simulink library "libAeroLookUpTables"  (R2020b)
settings: Solver=VariableStepAuto  StartTime=0.0  StopTime=10.0  RelTol=1e-3
undefined symbols (not defined in the file): data, table
settings Model: Creator=caatay  LastModifiedBy=caatay

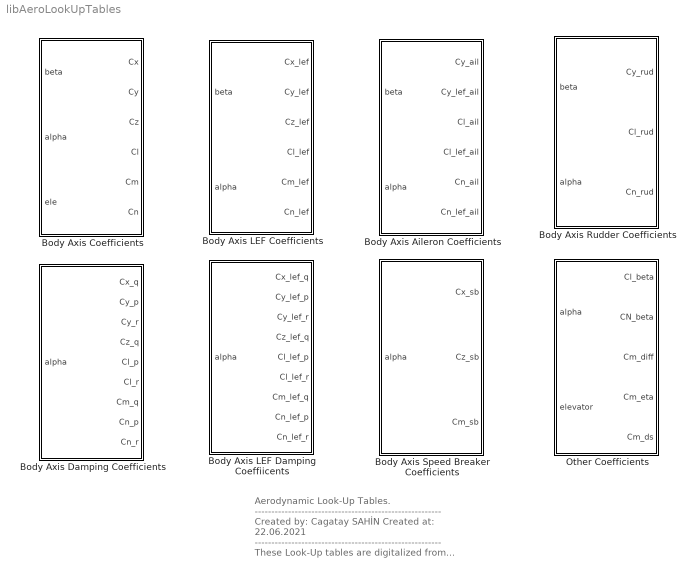
== system libAeroLookUpTables ==
  note: Aerodynamic Look-Up Tables.
      | --------------------------------------------------------
      | Created by: Cagatay SAHİN
      | Created at: 22.06.2021
      | --------------------------------------------------------
      | These Look-Up tables are digitalized from
      | Nguyen's NASA works.
      | The reference article can be found in
      | "references folder".
      | --------------------------------------------------------
      | for question:
      | cagataysahin44@gmail.com
  Body Axis Aileron Coefficients : Subsystem  mask(Aerodynamic Model - Look-Up Tables - Body Axis Aileron Aerodynamic Data){data=data}
      mask prompts: data "Aerodynamic Look-Up Table Data"
      mask help: 2-D Body axis aerodynamic look-up tables, effect on aileron deflection, to obtain that aerodynamic coefficients with using linear interpolation methods.
      mask Help:
      | This block calculates body axis aileron aerodynamic coefficient with using interpolation method.
      | According to reference, all look-up tables are 2-dimension.
      | -------------------------------------------------------------------------------------------------------------------------------------------------
      | Inputs of this block set are;
      | 	alpha = Angle of attack value that comes from equation of motion or frame transformation. [deg]
      | 	beta = Sideslip angle value that comes from equation of motion or frame transformation. [deg]
      | Output of this block set is;
      | 	C_{i_{ail}} = Body axis coefficients for instance Cx_rud, Cy_rud Cz_rud... .
      | -------------------------------------------------------------------------------------------------------------------------------------------------
      | Look-up tables are obtained from Nguyen's work. Reference can be found in "literature" subfolder.
      | For question: "cagataysahin44@gmail.com"
      mask Display:
      | port_label('input',1,'\beta','texmode','on');
      | port_label('input',2,'\alpha','texmode','on');
      | 
      | port_label('output',1,'C_{y_{ail}}','texmode','on');
      | port_label('output',2,'C_{y_{lef_{ail}}}','texmode','on');
      | port_label('output',3,'C_{l_{ail}}','texmode','on');
      | port_label('output',4,'C_{l_{lef_{ail}}}','texmode','on');
      | port_label('output',5,'C_{n_{ail}}','texmode','on');
      | port_label('output',6,'C_{n_{lef_{ail}}}','texmode','on');
  Body Axis Coefficients : Subsystem  mask(Aerodynamic Model - Look-Up Tables - Body Axis Aerodynamic Data){data=data}
      mask prompts: data "Aerodynamic Look-up Table Data"
      mask help: 3-D body axis aerodynamic look-up tables to obtain body axis aerodynamic coefficients with using interpolation method.
      mask Help:
      | This block calculates body axis aerodynamic coefficient with using interpolation method.
      | According to reference, all look-up tables are 3-dimension except "CY".
      | -------------------------------------------------------------------------------------------------------------------------------------------------
      | Inputs of this block set are;
      | 	alpha = Angle of attack value that comes from equation of motion or frame transformation. [deg]
      | 	beta = Sideslip angle value that comes from equation of motion or frame transformation. [deg]
      | 	elevator = Actuated elevator deflection value that comes from actuator. [deg]
      | Output of this block set is;
      | 	C_{i} = Body axis coefficients for instance Cx, Cy, Cz ... .
      | -------------------------------------------------------------------------------------------------------------------------------------------------
      | Look-up tables are obtained from Nguyen's work. Reference can be found in "literature" subfolder.
      | For question: "cagataysahin44@gmail.com"
      mask Display:
      | port_label('input',1,'\beta','texmode','on');
      | port_label('input',2,'\alpha','texmode','on');
      | port_label('input',3,'\delta_{el}','texmode','on');
      | 
      | port_label('output',1,'C_{x}','texmode','on');
      | port_label('output',2,'C_{y}','texmode','on');
      | port_label('output',3,'C_{z}','texmode','on');
      | port_label('output',4,'C_{l}','texmode','on');
      | port_label('output',5,'C_{m}','texmode','on');
      | port_label('output',6,'C_{n}','texmode','on');
  Body Axis Damping Coefficients : Subsystem  mask(Aerodynamic Model - Look-Up Tables - Body Axis Damping Aerodynamic Data){data=data}
      mask prompts: data "Aerodynamic Look-Up Table Data"
      mask help: 1-D Body axis damping aerodynamic look-up tables to obtain body axis damping aerodynamic coefficients with using interpolation method.
      mask Help:
      | This block calculates body axis aerodynamic coefficient with using interpolation method.
      | According to reference, all look-up tables are 1-dimension
      | -------------------------------------------------------------------------------------------------------------------------------------------------
      | Inputs of this block set are;
      | 	alpha = Angle of attack value that comes from equation of motion or frame transformation. [deg]
      | Output of this block set is;
      | 	C_{i_{j}} = Body axis damping coefficients for instance Cx_q, Cy_p, Cz_q ... .
      | -------------------------------------------------------------------------------------------------------------------------------------------------
      | Look-up tables are obtained from Nguyen's work. Reference can be found in "literature" subfolder.
      | For question: "cagataysahin44@gmail.com"
      mask Display:
      | port_label('input',1,'\alpha','texmode','on');
      | 
      | 
      | port_label('output',1,'C_{x_{q}}','texmode','on');
      | port_label('output',2,'C_{y_{p}}','texmode','on');
      | port_label('output',3,'C_{y_{r}}','texmode','on');
      | port_label('output',4,'C_{z_{q}}','texmode','on');
      | port_label('output',5,'C_{l_{p}}','texmode','on');
      | port_label('output',6,'C_{l_{r}}','texmode','on');
      | port_label('output',7,'C_{m_{q}}','texmode','on');
      | port_label('output',8,'C_{n_{p}}','texmode','on');
      | port_label('output',9,'C_{n_{r}}','texmode','on');
  Body Axis LEF Damping Coeffiicents : Subsystem  mask(Aerodynamic Model - Look-Up Tables - Body Axis LEF Damping Aerodynamic Data){data=data}
      mask prompts: data "Aerodynamic Look-Up Table Data"
      mask help: 1-D Body axis damping aerodynamic look-up tables, effect on leading edge flap deflections, to obtain that aerodynamic coefficient with using interpolation method.
      mask Help:
      | This block calculates body axis LEF aerodynamic coefficient with using interpolation method.
      | According to reference, all look-up tables are 1-dimension
      | -------------------------------------------------------------------------------------------------------------------------------------------------
      | Inputs of this block set are;
      | 	alpha = Angle of attack value that comes from equation of motion or frame transformation. [deg]
      | Output of this block set is;
      | 	C_{i_lef_{j}} = Body axis damping coefficients for instance Cx_lef_q, Cy_lef_p, Cz_lef_q ... .
      | -------------------------------------------------------------------------------------------------------------------------------------------------
      | Look-up tables are obtained from Nguyen's work. Reference can be found in "literature" subfolder.
      | For question: "cagataysahin44@gmail.com"
      mask Display:
      | port_label('input',1,'\alpha','texmode','on');
      | 
      | 
      | port_label('output',1,'C_{x_{lef}_{q}}','texmode','on');
      | port_label('output',2,'C_{y_{lef}_{p}}','texmode','on');
      | port_label('output',3,'C_{y_{lef}_{r}}','texmode','on');
      | port_label('output',4,'C_{z_{lef}_{q}}','texmode','on');
      | port_label('output',5,'C_{l_{lef}_{p}}','texmode','on');
      | port_label('output',6,'C_{l_{lef}_{r}}','texmode','on');
      | port_label('output',7,'C_{m_{lef}_{q}}','texmode','on');
      | port_label('output',8,'C_{n_{lef}_{p}}','texmode','on');
      | port_label('output',9,'C_{n_{lef}_{r}}','texmode','on');
  Body Axis LEF Coefficients : Subsystem  mask(Aerodynamic Model - Look-Up Tables - Body Axis Leading Edge Flap Aerodynamic Data){data=data}
      mask prompts: data "Aerodynamic Look-up Table Data"
      mask help: 2-D body axis aerodynamic look-up tables, effect on leading edge flap deflection, to obtain that aerodynamic coefficients with using linear interpolation methods.
      mask Help:
      | This block calculates body axis LEF aerodynamic coefficient with using interpolation method.
      | According to reference, all look-up tables are 2-dimension.
      | -------------------------------------------------------------------------------------------------------------------------------------------------
      | Inputs of this block set are;
      | 	alpha = Angle of attack value that comes from equation of motion or frame transformation. [deg]
      | 	beta = Sideslip angle value that comes from equation of motion or frame transformation. [deg]
      | Output of this block set is;
      | 	C_{i_{lef}} = Body axis coefficients for instance Cx_lef, Cy_lef, Cz_lef ... .
      | -------------------------------------------------------------------------------------------------------------------------------------------------
      | Look-up tables are obtained from Nguyen's work. Reference can be found in "literature" subfolder.
      | For question: "cagataysahin44@gmail.com"
      mask Display:
      | port_label('input',1,'\beta','texmode','on');
      | port_label('input',2,'\alpha','texmode','on');
      | 
      | port_label('output',1,'C_{x_{lef}}','texmode','on');
      | port_label('output',2,'C_{y_{lef}}','texmode','on');
      | port_label('output',3,'C_{z_{lef}}','texmode','on');
      | port_label('output',4,'C_{l_{lef}}','texmode','on');
      | port_label('output',5,'C_{m_{lef}}','texmode','on');
      | port_label('output',6,'C_{n_{lef}}','texmode','on');
  Body Axis Rudder Coefficients : Subsystem  mask(Aerodynamic Model - Look-Up Tables - Body Axis Rudder Aerodynamic Data){data=data}
      mask prompts: data "Aerodynamic Look-up Table Data"
      mask help: 2-D Body axi aerodynamic look-up tables, effect on rudder deflection, to obtain that aerodynamic coefficients with using linear interpolation methods.
      mask Help:
      | This block calculates body axis rudder aerodynamic coefficient with using interpolation method.
      | According to reference, all look-up tables are 2-dimension.
      | -------------------------------------------------------------------------------------------------------------------------------------------------
      | Inputs of this block set are;
      | 	alpha = Angle of attack value that comes from equation of motion or frame transformation. [deg]
      | 	beta = Sideslip angle value that comes from equation of motion or frame transformation. [deg]
      | Output of this block set is;
      | 	C_{i_{rud}} = Body axis coefficients for instance Cx_rud, Cy_rud Cz_rud... .
      | -------------------------------------------------------------------------------------------------------------------------------------------------
      | Look-up tables are obtained from Nguyen's work. Reference can be found in "literature" subfolder.
      | For question: "cagataysahin44@gmail.com"
      mask Display:
      | port_label('input',1,'\beta','texmode','on');
      | port_label('input',2,'\alpha','texmode','on');
      | 
      | port_label('output',1,'C_{y_{rud}}','texmode','on');
      | port_label('output',2,'C_{l_{rud}}','texmode','on');
      | port_label('output',3,'C_{n_{rud}}','texmode','on');
  Body Axis Speed Breaker Coefficients : Subsystem  mask(Aerodynamic Model - Look-Up Tables - Body Axis Speed Breaker Aerodynamic Data){data=data}
      mask prompts: data "Aerodynamic Look-Up Table Data"
      mask help: 2-D Body axis aerodynamic look-up tables, effect on speed breaker deflection, to obtain that aerodynamic coefficients with using linear interpolation methods.
      mask Help:
      | This block calculates body axis sb aerodynamic coefficient with using interpolation method.
      | According to reference, all look-up tables are 2-dimension.
      | -------------------------------------------------------------------------------------------------------------------------------------------------
      | Inputs of this block set are;
      | 	alpha = Angle of attack value that comes from equation of motion or frame transformation. [deg]
      | Output of this block set is;
      | 	C_{i_{rud}} = Body axis coefficients for instance Cx_rud, Cy_rud Cz_rud... .
      | -------------------------------------------------------------------------------------------------------------------------------------------------
      | Look-up tables are obtained from Nguyen's work. Reference can be found in "literature" subfolder.
      | For question: "cagataysahin44@gmail.com"
      mask Display:
      | port_label('input',1,'\alpha','texmode','on');
      | 
      | port_label('output',1,'C_{x_{sb}}','texmode','on');
      | port_label('output',2,'C_{z_{sb}}','texmode','on');
      | port_label('output',3,'C_{m_{sb}}','texmode','on');
  Other Coefficients : Subsystem  mask(Aerodynamic Model - Look-Up Tables - Other Aerodynamic Data){data=data}
      mask prompts: data "Aerodynamic Look-Up Table Data"
      mask help: 1-D Body axis aerodynamic look-up tables, which the remaning and uncategorized tables, to obtain aerodynamic coefficient with using interpolation method.
      mask Help:
      | This block calculates other/remaining aerodynamic coefficient with using interpolation method.
      | According to reference, all look-up tables are 1-dimension.
      | -------------------------------------------------------------------------------------------------------------------------------------------------
      | Inputs of this block set are;
      | 	alpha = Angle of attack value that comes from equation of motion or frame transformation. [deg]
      | 	elevator = Actuated elevator deflection angle value that comes from actuator. [deg]
      | Output of this block set is;
      | 	C_{i_{xx}} = Body axis coefficients for instance Cl_beta, Cn_beta, Cz_rud... .
      | -------------------------------------------------------------------------------------------------------------------------------------------------
      | Look-up tables are obtained from Nguyen's work. Reference can be found in "literature" subfolder.
      | For question: "cagataysahin44@gmail.com"
      mask Display:
      | port_label('input',1,'\alpha','texmode','on');
      | port_label('input',2,'\delta_{ele}','texmode','on');
      | 
      | port_label('output',1,'C_{l_{beta}}','texmode','on');
      | port_label('output',2,'C_{n_{beta}}','texmode','on');
      | port_label('output',3,'C_{m_{diff}}','texmode','on');
      | port_label('output',4,'C_{m_{eta}}','texmode','on');
      | port_label('output',5,'C_{m_{s}}','texmode','on');

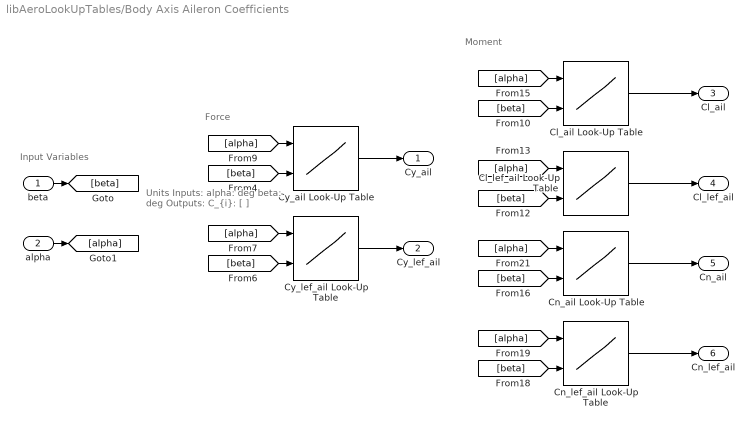
== system libAeroLookUpTables/Body Axis Aileron Coefficients ==
  note: Units
      | Inputs:
      | alpha: deg
      | beta: deg
      | Outputs:
      | C_{i}: [ ]
  note: Input Variables
  note: Force
  note: Moment
  beta : Inport
  alpha : Inport  Port=2
  Cl_ail Look-Up Table : Lookup_n-D  BreakpointsForDimension1=data.aero.coeffs.table.refSignals.alphaLong  BreakpointsForDimension2=data.aero.coeffs.table.refSignals.beta  Table=data.aero.coeffs.table.roll.Cl_ail  InternalRulePriority=Speed  RndMeth=Simplest  InputSameDT=on
      settings: InputPortMap=u0,u1
  Cl_lef_ail Look-Up Table : Lookup_n-D  BreakpointsForDimension1=data.aero.coeffs.table.refSignals.alphaShort  BreakpointsForDimension2=data.aero.coeffs.table.refSignals.beta  Table=data.aero.coeffs.table.roll.Cl_lef_ail  InternalRulePriority=Speed  RndMeth=Simplest  InputSameDT=on
      settings: InputPortMap=u0,u1
  Cn_ail Look-Up Table : Lookup_n-D  BreakpointsForDimension1=data.aero.coeffs.table.refSignals.alphaLong  BreakpointsForDimension2=data.aero.coeffs.table.refSignals.beta  Table=data.aero.coeffs.table.yaw.Cn_ail  InternalRulePriority=Speed  RndMeth=Simplest  InputSameDT=on
      settings: InputPortMap=u0,u1
  Cn_lef_ail Look-Up Table : Lookup_n-D  BreakpointsForDimension1=data.aero.coeffs.table.refSignals.alphaShort  BreakpointsForDimension2=data.aero.coeffs.table.refSignals.beta  Table=data.aero.coeffs.table.yaw.Cn_lef_ail  InternalRulePriority=Speed  RndMeth=Simplest  InputSameDT=on
      settings: InputPortMap=u0,u1
  Cy_ail Look-Up Table : Lookup_n-D  BreakpointsForDimension1=data.aero.coeffs.table.refSignals.alphaLong  BreakpointsForDimension2=data.aero.coeffs.table.refSignals.beta  Table=data.aero.coeffs.table.yaxis.Cy_ail  InternalRulePriority=Speed  RndMeth=Simplest  InputSameDT=on
      settings: InputPortMap=u0,u1
  Cy_lef_ail Look-Up Table : Lookup_n-D  BreakpointsForDimension1=data.aero.coeffs.table.refSignals.alphaShort  BreakpointsForDimension2=data.aero.coeffs.table.refSignals.beta  Table=data.aero.coeffs.table.yaxis.Cy_lef_ail  InternalRulePriority=Speed  RndMeth=Simplest  InputSameDT=on
      settings: InputPortMap=u0,u1
  Cy_ail : Outport  VectorParamsAs1DForOutWhenUnconnected=off
  Cy_lef_ail : Outport  Port=2  VectorParamsAs1DForOutWhenUnconnected=off
  Cl_ail : Outport  Port=3  VectorParamsAs1DForOutWhenUnconnected=off
  Cl_lef_ail : Outport  Port=4  VectorParamsAs1DForOutWhenUnconnected=off
  Cn_ail : Outport  Port=5  VectorParamsAs1DForOutWhenUnconnected=off
  Cn_lef_ail : Outport  Port=6  VectorParamsAs1DForOutWhenUnconnected=off
  wires:
  Cn_lef_ail Look-Up Table/1 -> Cn_lef_ail/1
  Cl_lef_ail Look-Up Table/1 -> Cl_lef_ail/1
  Cy_lef_ail Look-Up Table/1 -> Cy_lef_ail/1
  beta/1 -> [beta]
  alpha/1 -> [alpha]
  Cy_ail Look-Up Table/1 -> Cy_ail/1
  Cn_ail Look-Up Table/1 -> Cn_ail/1
  Cl_ail Look-Up Table/1 -> Cl_ail/1
  [beta] -> Cy_lef_ail Look-Up Table/2
  [alpha] -> Cy_lef_ail Look-Up Table/1
  [beta] -> Cy_ail Look-Up Table/2
  [alpha] -> Cy_ail Look-Up Table/1
  [alpha] -> Cl_ail Look-Up Table/1
  [beta] -> Cl_ail Look-Up Table/2
  [alpha] -> Cl_lef_ail Look-Up Table/1
  [beta] -> Cl_lef_ail Look-Up Table/2
  [beta] -> Cn_ail Look-Up Table/2
  [alpha] -> Cn_ail Look-Up Table/1
  [alpha] -> Cn_lef_ail Look-Up Table/1
  [beta] -> Cn_lef_ail Look-Up Table/2

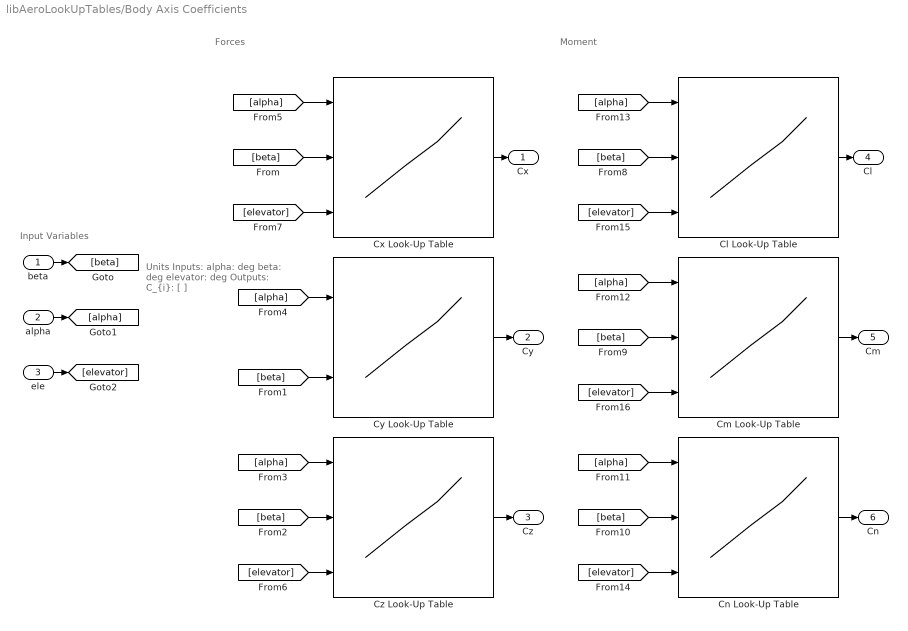
== system libAeroLookUpTables/Body Axis Coefficients ==
  note: Moment
  note: Input Variables
  note: Units
      | Inputs:
      | alpha: deg
      | beta: deg
      | elevator: deg
      | Outputs:
      | C_{i}: [ ]
  note: Forces
  beta : Inport
  alpha : Inport  Port=2
  ele : Inport  Port=3
  Cl Look-Up Table : Lookup_n-D  NumberOfTableDimensions=3  BreakpointsForDimension1=data.aero.coeffs.table.refSignals.alphaLong  BreakpointsForDimension2=data.aero.coeffs.table.refSignals.beta  BreakpointsForDimension3=data.aero.coeffs.table.refSignals.eleShort  Table=data.aero.coeffs.table.roll.Cl  InternalRulePriority=Speed  RndMeth=Simplest  InputSameDT=on
      settings: InputPortMap=u0,u1,u2
  Cm Look-Up Table : Lookup_n-D  NumberOfTableDimensions=3  BreakpointsForDimension1=data.aero.coeffs.table.refSignals.alphaLong  BreakpointsForDimension2=data.aero.coeffs.table.refSignals.beta  BreakpointsForDimension3=data.aero.coeffs.table.refSignals.eleLong  Table=data.aero.coeffs.table.pitch.Cm  InternalRulePriority=Speed  RndMeth=Simplest  InputSameDT=on
      settings: InputPortMap=u0,u1,u2
  Cn Look-Up Table : Lookup_n-D  NumberOfTableDimensions=3  BreakpointsForDimension1=data.aero.coeffs.table.refSignals.alphaLong  BreakpointsForDimension2=data.aero.coeffs.table.refSignals.beta  BreakpointsForDimension3=data.aero.coeffs.table.refSignals.eleShort  Table=data.aero.coeffs.table.yaw.Cn  InternalRulePriority=Speed  RndMeth=Simplest  InputSameDT=on
      settings: InputPortMap=u0,u1,u2
  Cx Look-Up Table : Lookup_n-D  NumberOfTableDimensions=3  BreakpointsForDimension1=data.aero.coeffs.table.refSignals.alphaLong  BreakpointsForDimension2=data.aero.coeffs.table.refSignals.beta  BreakpointsForDimension3=data.aero.coeffs.table.refSignals.eleLong  Table=data.aero.coeffs.table.xaxis.Cx  InternalRulePriority=Speed  RndMeth=Simplest  InputSameDT=on
      settings: InputPortMap=u0,u1,u2
  Cy Look-Up Table : Lookup_n-D  BreakpointsForDimension1=data.aero.coeffs.table.refSignals.alphaLong  BreakpointsForDimension2=data.aero.coeffs.table.refSignals.beta  BreakpointsForDimension3=table.aero.refSignal.eleLong  Table=data.aero.coeffs.table.yaxis.Cy  InternalRulePriority=Speed  RndMeth=Simplest  InputSameDT=on
      settings: InputPortMap=u0,u1
  Cz Look-Up Table : Lookup_n-D  NumberOfTableDimensions=3  BreakpointsForDimension1=data.aero.coeffs.table.refSignals.alphaLong  BreakpointsForDimension2=data.aero.coeffs.table.refSignals.beta  BreakpointsForDimension3=data.aero.coeffs.table.refSignals.eleLong  Table=data.aero.coeffs.table.zaxis.Cz  InternalRulePriority=Speed  RndMeth=Simplest  InputSameDT=on
      settings: InputPortMap=u0,u1,u2
  Cx : Outport  VectorParamsAs1DForOutWhenUnconnected=off
  Cy : Outport  Port=2  VectorParamsAs1DForOutWhenUnconnected=off
  Cz : Outport  Port=3  VectorParamsAs1DForOutWhenUnconnected=off
  Cl : Outport  Port=4  VectorParamsAs1DForOutWhenUnconnected=off
  Cm : Outport  Port=5  VectorParamsAs1DForOutWhenUnconnected=off
  Cn : Outport  Port=6  VectorParamsAs1DForOutWhenUnconnected=off
  wires:
  [elevator] -> Cm Look-Up Table/3
  [elevator] -> Cl Look-Up Table/3
  [elevator] -> Cn Look-Up Table/3
  Cn Look-Up Table/1 -> Cn/1
  Cm Look-Up Table/1 -> Cm/1
  Cl Look-Up Table/1 -> Cl/1
  [elevator] -> Cx Look-Up Table/3
  [elevator] -> Cz Look-Up Table/3
  Cy Look-Up Table/1 -> Cy/1
  Cz Look-Up Table/1 -> Cz/1
  ele/1 -> [elevator]
  beta/1 -> [beta]
  alpha/1 -> [alpha]
  Cx Look-Up Table/1 -> Cx/1
  [beta] -> Cx Look-Up Table/2
  [alpha] -> Cx Look-Up Table/1
  [alpha] -> Cy Look-Up Table/1
  [beta] -> Cy Look-Up Table/2
  [alpha] -> Cz Look-Up Table/1
  [beta] -> Cz Look-Up Table/2
  [alpha] -> Cl Look-Up Table/1
  [beta] -> Cl Look-Up Table/2
  [alpha] -> Cn Look-Up Table/1
  [beta] -> Cn Look-Up Table/2
  [beta] -> Cm Look-Up Table/2
  [alpha] -> Cm Look-Up Table/1

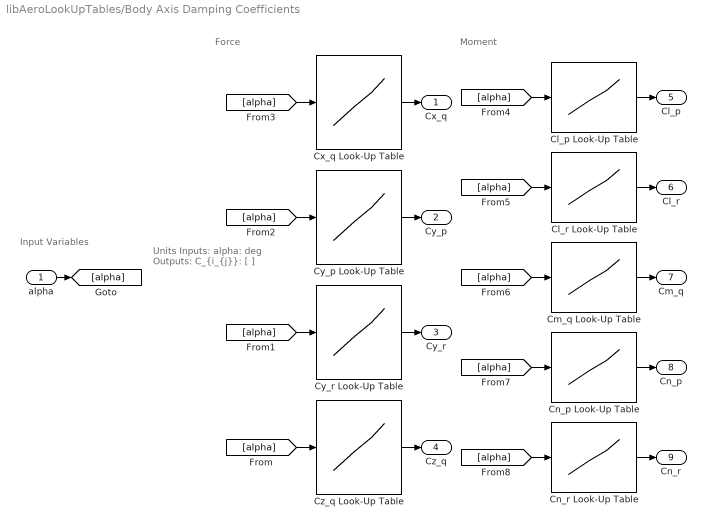
== system libAeroLookUpTables/Body Axis Damping Coefficients ==
  note: Units
      | Inputs:
      | alpha: deg
      | Outputs:
      | C_{i_{j}}: [ ]
  note: Input Variables
  note: Force
  note: Moment
  alpha : Inport
  Cl_p Look-Up Table : Lookup_n-D  NumberOfTableDimensions=1  BreakpointsForDimension1=data.aero.coeffs.table.refSignals.alphaLong  Table=data.aero.coeffs.table.roll.Cl_p  InternalRulePriority=Speed  RndMeth=Simplest  InputSameDT=on
  Cl_r Look-Up Table : Lookup_n-D  NumberOfTableDimensions=1  BreakpointsForDimension1=data.aero.coeffs.table.refSignals.alphaLong  Table=data.aero.coeffs.table.roll.Cl_r  InternalRulePriority=Speed  RndMeth=Simplest  InputSameDT=on
  Cm_q Look-Up Table : Lookup_n-D  NumberOfTableDimensions=1  BreakpointsForDimension1=data.aero.coeffs.table.refSignals.alphaLong  Table=data.aero.coeffs.table.pitch.Cm_q  InternalRulePriority=Speed  RndMeth=Simplest  InputSameDT=on
  Cn_p Look-Up Table : Lookup_n-D  NumberOfTableDimensions=1  BreakpointsForDimension1=data.aero.coeffs.table.refSignals.alphaLong  Table=data.aero.coeffs.table.yaw.Cn_p  InternalRulePriority=Speed  RndMeth=Simplest  InputSameDT=on
  Cn_r Look-Up Table : Lookup_n-D  NumberOfTableDimensions=1  BreakpointsForDimension1=data.aero.coeffs.table.refSignals.alphaLong  Table=data.aero.coeffs.table.yaw.Cn_r  InternalRulePriority=Speed  RndMeth=Simplest  InputSameDT=on
  Cx_q Look-Up Table : Lookup_n-D  NumberOfTableDimensions=1  BreakpointsForDimension1=data.aero.coeffs.table.refSignals.alphaLong  Table=data.aero.coeffs.table.xaxis.Cx_q  InternalRulePriority=Speed  RndMeth=Simplest  InputSameDT=on
  Cy_p Look-Up Table : Lookup_n-D  NumberOfTableDimensions=1  BreakpointsForDimension1=data.aero.coeffs.table.refSignals.alphaLong  Table=data.aero.coeffs.table.yaxis.Cy_p  InternalRulePriority=Speed  RndMeth=Simplest  InputSameDT=on
  Cy_r Look-Up Table : Lookup_n-D  NumberOfTableDimensions=1  BreakpointsForDimension1=data.aero.coeffs.table.refSignals.alphaLong  Table=data.aero.coeffs.table.yaxis.Cy_r  InternalRulePriority=Speed  RndMeth=Simplest  InputSameDT=on
  Cz_q Look-Up Table : Lookup_n-D  NumberOfTableDimensions=1  BreakpointsForDimension1=data.aero.coeffs.table.refSignals.alphaLong  Table=data.aero.coeffs.table.zaxis.Cz_q  InternalRulePriority=Speed  RndMeth=Simplest  InputSameDT=on
  Cx_q : Outport  VectorParamsAs1DForOutWhenUnconnected=off
  Cy_p : Outport  Port=2  VectorParamsAs1DForOutWhenUnconnected=off
  Cy_r : Outport  Port=3  VectorParamsAs1DForOutWhenUnconnected=off
  Cz_q : Outport  Port=4  VectorParamsAs1DForOutWhenUnconnected=off
  Cl_p : Outport  Port=5  VectorParamsAs1DForOutWhenUnconnected=off
  Cl_r : Outport  Port=6  VectorParamsAs1DForOutWhenUnconnected=off
  Cm_q : Outport  Port=7  VectorParamsAs1DForOutWhenUnconnected=off
  Cn_p : Outport  Port=8  VectorParamsAs1DForOutWhenUnconnected=off
  Cn_r : Outport  Port=9  VectorParamsAs1DForOutWhenUnconnected=off
  wires:
  Cn_r Look-Up Table/1 -> Cn_r/1
  Cn_p Look-Up Table/1 -> Cn_p/1
  Cm_q Look-Up Table/1 -> Cm_q/1
  Cl_r Look-Up Table/1 -> Cl_r/1
  Cl_p Look-Up Table/1 -> Cl_p/1
  [alpha] -> Cn_r Look-Up Table/1
  [alpha] -> Cn_p Look-Up Table/1
  [alpha] -> Cm_q Look-Up Table/1
  [alpha] -> Cl_r Look-Up Table/1
  [alpha] -> Cl_p Look-Up Table/1
  Cz_q Look-Up Table/1 -> Cz_q/1
  Cy_r Look-Up Table/1 -> Cy_r/1
  Cy_p Look-Up Table/1 -> Cy_p/1
  Cx_q Look-Up Table/1 -> Cx_q/1
  [alpha] -> Cx_q Look-Up Table/1
  [alpha] -> Cy_p Look-Up Table/1
  [alpha] -> Cy_r Look-Up Table/1
  [alpha] -> Cz_q Look-Up Table/1
  alpha/1 -> [alpha]

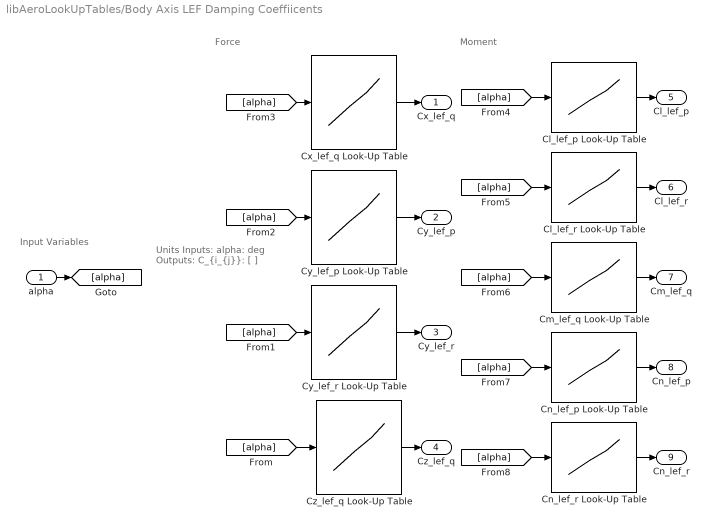
== system libAeroLookUpTables/Body Axis LEF Damping Coeffiicents ==
  note: Input Variables
  note: Units
      | Inputs:
      | alpha: deg
      | Outputs:
      | C_{i_{j}}: [ ]
  note: Force
  note: Moment
  alpha : Inport
  Cl_lef_p Look-Up Table : Lookup_n-D  NumberOfTableDimensions=1  BreakpointsForDimension1=data.aero.coeffs.table.refSignals.alphaShort  Table=data.aero.coeffs.table.roll.Cl_lef_p  InternalRulePriority=Speed  RndMeth=Simplest  InputSameDT=on
  Cl_lef_r Look-Up Table : Lookup_n-D  NumberOfTableDimensions=1  BreakpointsForDimension1=data.aero.coeffs.table.refSignals.alphaShort  Table=data.aero.coeffs.table.roll.Cl_lef_r  InternalRulePriority=Speed  RndMeth=Simplest  InputSameDT=on
  Cm_lef_q Look-Up Table : Lookup_n-D  NumberOfTableDimensions=1  BreakpointsForDimension1=data.aero.coeffs.table.refSignals.alphaShort  Table=data.aero.coeffs.table.pitch.Cm_lef_q  InternalRulePriority=Speed  RndMeth=Simplest  InputSameDT=on
  Cn_lef_p Look-Up Table : Lookup_n-D  NumberOfTableDimensions=1  BreakpointsForDimension1=data.aero.coeffs.table.refSignals.alphaShort  Table=data.aero.coeffs.table.yaw.Cn_lef_p  InternalRulePriority=Speed  RndMeth=Simplest  InputSameDT=on
  Cn_lef_r Look-Up Table : Lookup_n-D  NumberOfTableDimensions=1  BreakpointsForDimension1=data.aero.coeffs.table.refSignals.alphaShort  Table=data.aero.coeffs.table.yaw.Cn_lef_r  InternalRulePriority=Speed  RndMeth=Simplest  InputSameDT=on
  Cx_lef_q Look-Up Table : Lookup_n-D  NumberOfTableDimensions=1  BreakpointsForDimension1=data.aero.coeffs.table.refSignals.alphaShort  Table=data.aero.coeffs.table.xaxis.Cx_lef_q  InternalRulePriority=Speed  RndMeth=Simplest  InputSameDT=on
  Cy_lef_p Look-Up Table : Lookup_n-D  NumberOfTableDimensions=1  BreakpointsForDimension1=data.aero.coeffs.table.refSignals.alphaShort  Table=data.aero.coeffs.table.yaxis.Cy_lef_p  InternalRulePriority=Speed  RndMeth=Simplest  InputSameDT=on
  Cy_lef_r Look-Up Table : Lookup_n-D  NumberOfTableDimensions=1  BreakpointsForDimension1=data.aero.coeffs.table.refSignals.alphaShort  Table=data.aero.coeffs.table.yaxis.Cy_lef_r  InternalRulePriority=Speed  RndMeth=Simplest  InputSameDT=on
  Cz_lef_q Look-Up Table : Lookup_n-D  NumberOfTableDimensions=1  BreakpointsForDimension1=data.aero.coeffs.table.refSignals.alphaShort  Table=data.aero.coeffs.table.zaxis.Cz_lef_q  InternalRulePriority=Speed  RndMeth=Simplest  InputSameDT=on
  Cx_lef_q : Outport  VectorParamsAs1DForOutWhenUnconnected=off
  Cy_lef_p : Outport  Port=2  VectorParamsAs1DForOutWhenUnconnected=off
  Cy_lef_r : Outport  Port=3  VectorParamsAs1DForOutWhenUnconnected=off
  Cz_lef_q : Outport  Port=4  VectorParamsAs1DForOutWhenUnconnected=off
  Cl_lef_p : Outport  Port=5  VectorParamsAs1DForOutWhenUnconnected=off
  Cl_lef_r : Outport  Port=6  VectorParamsAs1DForOutWhenUnconnected=off
  Cm_lef_q : Outport  Port=7  VectorParamsAs1DForOutWhenUnconnected=off
  Cn_lef_p : Outport  Port=8  VectorParamsAs1DForOutWhenUnconnected=off
  Cn_lef_r : Outport  Port=9  VectorParamsAs1DForOutWhenUnconnected=off
  wires:
  [alpha] -> Cm_lef_q Look-Up Table/1
  Cm_lef_q Look-Up Table/1 -> Cm_lef_q/1
  Cl_lef_p Look-Up Table/1 -> Cl_lef_p/1
  Cl_lef_r Look-Up Table/1 -> Cl_lef_r/1
  [alpha] -> Cl_lef_r Look-Up Table/1
  Cn_lef_p Look-Up Table/1 -> Cn_lef_p/1
  [alpha] -> Cn_lef_p Look-Up Table/1
  [alpha] -> Cl_lef_p Look-Up Table/1
  [alpha] -> Cz_lef_q Look-Up Table/1
  Cn_lef_r Look-Up Table/1 -> Cn_lef_r/1
  Cz_lef_q Look-Up Table/1 -> Cz_lef_q/1
  Cy_lef_r Look-Up Table/1 -> Cy_lef_r/1
  [alpha] -> Cx_lef_q Look-Up Table/1
  [alpha] -> Cy_lef_p Look-Up Table/1
  [alpha] -> Cn_lef_r Look-Up Table/1
  Cx_lef_q Look-Up Table/1 -> Cx_lef_q/1
  [alpha] -> Cy_lef_r Look-Up Table/1
  alpha/1 -> [alpha]
  Cy_lef_p Look-Up Table/1 -> Cy_lef_p/1

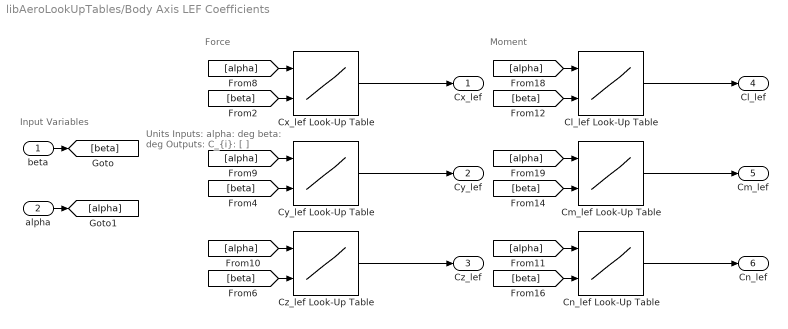
== system libAeroLookUpTables/Body Axis LEF Coefficients ==
  note: Moment
  note: Units
      | Inputs:
      | alpha: deg
      | beta: deg
      | Outputs:
      | C_{i}: [ ]
  note: Input Variables
  note: Force
  beta : Inport
  alpha : Inport  Port=2
  Cl_lef Look-Up Table : Lookup_n-D  BreakpointsForDimension1=data.aero.coeffs.table.refSignals.alphaShort  BreakpointsForDimension2=data.aero.coeffs.table.refSignals.beta  Table=data.aero.coeffs.table.roll.Cl_lef  InternalRulePriority=Speed  RndMeth=Simplest  InputSameDT=on
      settings: InputPortMap=u0,u1
  Cm_lef Look-Up Table : Lookup_n-D  BreakpointsForDimension1=data.aero.coeffs.table.refSignals.alphaShort  BreakpointsForDimension2=data.aero.coeffs.table.refSignals.beta  Table=data.aero.coeffs.table.pitch.Cm_lef  InternalRulePriority=Speed  RndMeth=Simplest  InputSameDT=on
      settings: InputPortMap=u0,u1
  Cn_lef Look-Up Table : Lookup_n-D  BreakpointsForDimension1=data.aero.coeffs.table.refSignals.alphaShort  BreakpointsForDimension2=data.aero.coeffs.table.refSignals.beta  Table=data.aero.coeffs.table.yaw.Cn_lef  InternalRulePriority=Speed  RndMeth=Simplest  InputSameDT=on
      settings: InputPortMap=u0,u1
  Cx_lef Look-Up Table : Lookup_n-D  BreakpointsForDimension1=data.aero.coeffs.table.refSignals.alphaShort  BreakpointsForDimension2=data.aero.coeffs.table.refSignals.beta  Table=data.aero.coeffs.table.xaxis.Cx_lef  InternalRulePriority=Speed  RndMeth=Simplest  InputSameDT=on
      settings: InputPortMap=u0,u1
  Cy_lef Look-Up Table : Lookup_n-D  BreakpointsForDimension1=data.aero.coeffs.table.refSignals.alphaShort  BreakpointsForDimension2=data.aero.coeffs.table.refSignals.beta  Table=data.aero.coeffs.table.yaxis.Cy_lef  InternalRulePriority=Speed  RndMeth=Simplest  InputSameDT=on
      settings: InputPortMap=u0,u1
  Cz_lef Look-Up Table : Lookup_n-D  BreakpointsForDimension1=data.aero.coeffs.table.refSignals.alphaShort  BreakpointsForDimension2=data.aero.coeffs.table.refSignals.beta  Table=data.aero.coeffs.table.zaxis.Cz_lef  InternalRulePriority=Speed  RndMeth=Simplest  InputSameDT=on
      settings: InputPortMap=u0,u1
  Cx_lef : Outport  VectorParamsAs1DForOutWhenUnconnected=off
  Cy_lef : Outport  Port=2  VectorParamsAs1DForOutWhenUnconnected=off
  Cz_lef : Outport  Port=3  VectorParamsAs1DForOutWhenUnconnected=off
  Cl_lef : Outport  Port=4  VectorParamsAs1DForOutWhenUnconnected=off
  Cm_lef : Outport  Port=5  VectorParamsAs1DForOutWhenUnconnected=off
  Cn_lef : Outport  Port=6  VectorParamsAs1DForOutWhenUnconnected=off
  wires:
  Cn_lef Look-Up Table/1 -> Cn_lef/1
  Cl_lef Look-Up Table/1 -> Cl_lef/1
  Cm_lef Look-Up Table/1 -> Cm_lef/1
  Cz_lef Look-Up Table/1 -> Cz_lef/1
  Cy_lef Look-Up Table/1 -> Cy_lef/1
  Cx_lef Look-Up Table/1 -> Cx_lef/1
  beta/1 -> [beta]
  alpha/1 -> [alpha]
  [beta] -> Cx_lef Look-Up Table/2
  [alpha] -> Cx_lef Look-Up Table/1
  [alpha] -> Cy_lef Look-Up Table/1
  [beta] -> Cy_lef Look-Up Table/2
  [alpha] -> Cz_lef Look-Up Table/1
  [beta] -> Cz_lef Look-Up Table/2
  [alpha] -> Cn_lef Look-Up Table/1
  [beta] -> Cn_lef Look-Up Table/2
  [beta] -> Cm_lef Look-Up Table/2
  [alpha] -> Cm_lef Look-Up Table/1
  [beta] -> Cl_lef Look-Up Table/2
  [alpha] -> Cl_lef Look-Up Table/1

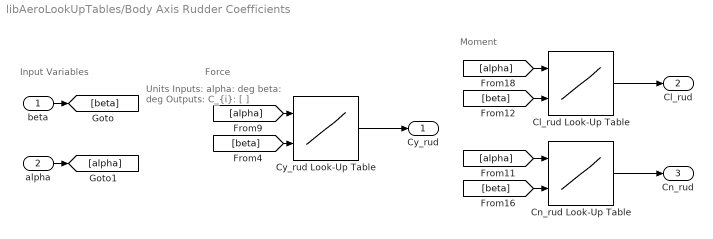
== system libAeroLookUpTables/Body Axis Rudder Coefficients ==
  note: Moment
  note: Input Variables
  note: Units
      | Inputs:
      | alpha: deg
      | beta: deg
      | Outputs:
      | C_{i}: [ ]
  note: Force
  beta : Inport
  alpha : Inport  Port=2
  Cl_rud Look-Up Table : Lookup_n-D  BreakpointsForDimension1=data.aero.coeffs.table.refSignals.alphaLong  BreakpointsForDimension2=data.aero.coeffs.table.refSignals.beta  Table=data.aero.coeffs.table.roll.Cl_rud  InternalRulePriority=Speed  RndMeth=Simplest  InputSameDT=on
      settings: InputPortMap=u0,u1
  Cn_rud Look-Up Table : Lookup_n-D  BreakpointsForDimension1=data.aero.coeffs.table.refSignals.alphaLong  BreakpointsForDimension2=data.aero.coeffs.table.refSignals.beta  Table=data.aero.coeffs.table.yaw.Cn_rud  InternalRulePriority=Speed  RndMeth=Simplest  InputSameDT=on
      settings: InputPortMap=u0,u1
  Cy_rud Look-Up Table : Lookup_n-D  BreakpointsForDimension1=data.aero.coeffs.table.refSignals.alphaLong  BreakpointsForDimension2=data.aero.coeffs.table.refSignals.beta  Table=data.aero.coeffs.table.yaxis.Cy_rud  InternalRulePriority=Speed  RndMeth=Simplest  InputSameDT=on
      settings: InputPortMap=u0,u1
  Cy_rud : Outport  VectorParamsAs1DForOutWhenUnconnected=off
  Cl_rud : Outport  Port=2  VectorParamsAs1DForOutWhenUnconnected=off
  Cn_rud : Outport  Port=3  VectorParamsAs1DForOutWhenUnconnected=off
  wires:
  beta/1 -> [beta]
  Cl_rud Look-Up Table/1 -> Cl_rud/1
  Cn_rud Look-Up Table/1 -> Cn_rud/1
  alpha/1 -> [alpha]
  Cy_rud Look-Up Table/1 -> Cy_rud/1
  [beta] -> Cy_rud Look-Up Table/2
  [alpha] -> Cy_rud Look-Up Table/1
  [alpha] -> Cl_rud Look-Up Table/1
  [beta] -> Cl_rud Look-Up Table/2
  [alpha] -> Cn_rud Look-Up Table/1
  [beta] -> Cn_rud Look-Up Table/2

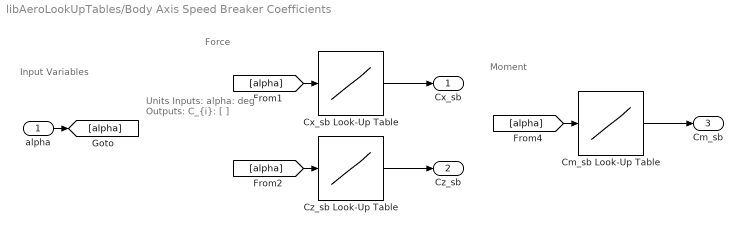
== system libAeroLookUpTables/Body Axis Speed Breaker Coefficients ==
  note: Force
  note: Input Variables
  note: Units
      | Inputs:
      | alpha: deg
      | Outputs:
      | C_{i}: [ ]
  note: Moment
  alpha : Inport
  Cm_sb Look-Up Table : Lookup_n-D  NumberOfTableDimensions=1  BreakpointsForDimension1=data.aero.coeffs.table.refSignals.alphaLong  BreakpointsForDimension2=data.aero.coeffs.table.refSignals.beta  Table=data.aero.coeffs.table.pitch.Cm_sb  InternalRulePriority=Speed  RndMeth=Simplest  InputSameDT=on
  Cx_sb Look-Up Table : Lookup_n-D  NumberOfTableDimensions=1  BreakpointsForDimension1=data.aero.coeffs.table.refSignals.alphaLong  BreakpointsForDimension2=data.aero.coeffs.table.refSignals.beta  Table=data.aero.coeffs.table.xaxis.Cx_sb  InternalRulePriority=Speed  RndMeth=Simplest  InputSameDT=on
  Cz_sb Look-Up Table : Lookup_n-D  NumberOfTableDimensions=1  BreakpointsForDimension1=data.aero.coeffs.table.refSignals.alphaLong  BreakpointsForDimension2=data.aero.coeffs.table.refSignals.beta  Table=data.aero.coeffs.table.zaxis.Cz_sb  InternalRulePriority=Speed  RndMeth=Simplest  InputSameDT=on
  Cx_sb : Outport  VectorParamsAs1DForOutWhenUnconnected=off
  Cz_sb : Outport  Port=2  VectorParamsAs1DForOutWhenUnconnected=off
  Cm_sb : Outport  Port=3  VectorParamsAs1DForOutWhenUnconnected=off
  wires:
  Cm_sb Look-Up Table/1 -> Cm_sb/1
  [alpha] -> Cm_sb Look-Up Table/1
  alpha/1 -> [alpha]
  Cx_sb Look-Up Table/1 -> Cx_sb/1
  [alpha] -> Cx_sb Look-Up Table/1
  [alpha] -> Cz_sb Look-Up Table/1
  Cz_sb Look-Up Table/1 -> Cz_sb/1

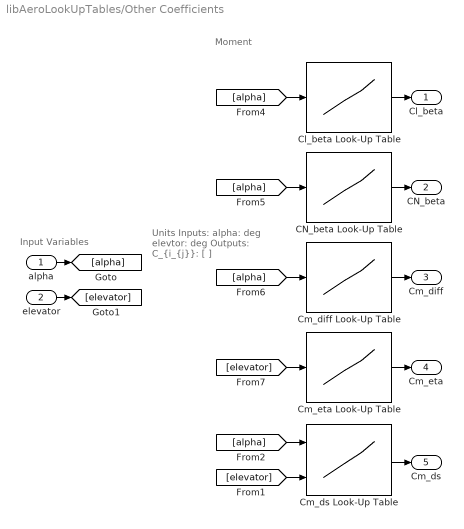
== system libAeroLookUpTables/Other Coefficients ==
  note: Input Variables
  note: Units
      | Inputs:
      | alpha: deg
      | elevtor: deg
      | Outputs:
      | C_{i_{j}}: [ ]
  note: Moment
  alpha : Inport
  elevator : Inport  Port=2
  CN_beta Look-Up Table : Lookup_n-D  NumberOfTableDimensions=1  BreakpointsForDimension1=data.aero.coeffs.table.refSignals.alphaLong  Table=data.aero.coeffs.table.yaw.Cn_beta  InternalRulePriority=Speed  RndMeth=Simplest  InputSameDT=on
  Cl_beta Look-Up Table : Lookup_n-D  NumberOfTableDimensions=1  BreakpointsForDimension1=data.aero.coeffs.table.refSignals.alphaLong  Table=data.aero.coeffs.table.roll.Cl_beta  InternalRulePriority=Speed  RndMeth=Simplest  InputSameDT=on
  Cm_diff Look-Up Table : Lookup_n-D  NumberOfTableDimensions=1  BreakpointsForDimension1=data.aero.coeffs.table.refSignals.alphaLong  Table=data.aero.coeffs.table.pitch.Cm_diff  InternalRulePriority=Speed  RndMeth=Simplest  InputSameDT=on
  Cm_ds Look-Up Table : Lookup_n-D  BreakpointsForDimension1=data.aero.coeffs.table.refSignals.alphaLong  BreakpointsForDimension2=data.aero.coeffs.table.refSignals.eleLongest  Table=data.aero.coeffs.table.pitch.Cm_ds  InternalRulePriority=Speed  RndMeth=Simplest  InputSameDT=on
      settings: InputPortMap=u0,u1
  Cm_eta Look-Up Table : Lookup_n-D  NumberOfTableDimensions=1  BreakpointsForDimension1=data.aero.coeffs.table.refSignals.eleLong  Table=data.aero.coeffs.table.pitch.Cm_eta  InternalRulePriority=Speed  RndMeth=Simplest  InputSameDT=on
  Cl_beta : Outport  VectorParamsAs1DForOutWhenUnconnected=off
  CN_beta : Outport  Port=2  VectorParamsAs1DForOutWhenUnconnected=off
  Cm_diff : Outport  Port=3  VectorParamsAs1DForOutWhenUnconnected=off
  Cm_eta : Outport  Port=4  VectorParamsAs1DForOutWhenUnconnected=off
  Cm_ds : Outport  Port=5  VectorParamsAs1DForOutWhenUnconnected=off
  wires:
  Cm_ds Look-Up Table/1 -> Cm_ds/1
  elevator/1 -> [elevator]
  [alpha] -> Cl_beta Look-Up Table/1
  Cl_beta Look-Up Table/1 -> Cl_beta/1
  alpha/1 -> [alpha]
  [alpha] -> CN_beta Look-Up Table/1
  [alpha] -> Cm_diff Look-Up Table/1
  [elevator] -> Cm_eta Look-Up Table/1
  Cm_diff Look-Up Table/1 -> Cm_diff/1
  CN_beta Look-Up Table/1 -> CN_beta/1
  Cm_eta Look-Up Table/1 -> Cm_eta/1
  [elevator] -> Cm_ds Look-Up Table/2
  [alpha] -> Cm_ds Look-Up Table/1
